simulink model "TST_EngBrk_ExhFlpCtl"  (R2016b)
settings: Solver=FixedStepDiscrete  StartTime=0.0  StopTime=simTime  FixedStep=sampleTime  RelTol=1e-3
values from neighbouring files (symbols this model uses):
  testCase = 1    [initTST_EngBrk_ExhFlpCtl_001.m]    (also in initTST_EngBrk_ExhFlpCtl_002.m = 2)
libraries: simulink x3
settings Model: Creator=WF305  LastModifiedBy=WF305
settings DebuggingCC: SignalRangeChecking=error

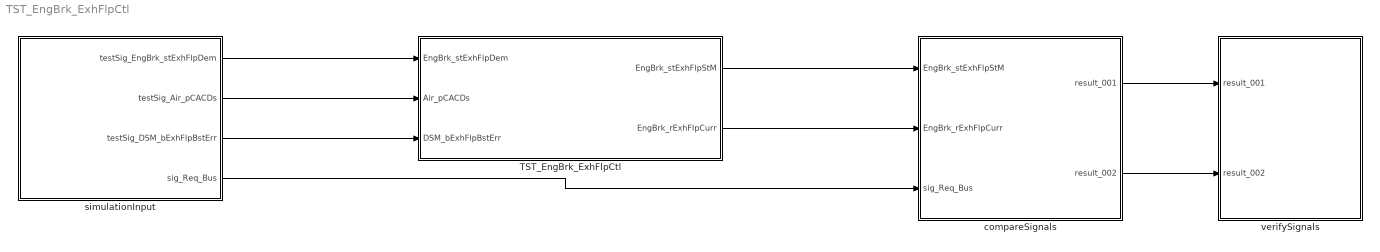
== system TST_EngBrk_ExhFlpCtl ==
  TST_EngBrk_ExhFlpCtl : Subsystem
  compareSignals : Subsystem
  simulationInput : Subsystem
  verifySignals : Subsystem
  wires:
  simulationInput/1(testSig_EngBrk_stExhFlpDem) -> TST_EngBrk_ExhFlpCtl/1(EngBrk_stExhFlpDem)
  simulationInput/2(testSig_Air_pCACDs) -> TST_EngBrk_ExhFlpCtl/2(Air_pCACDs)
  simulationInput/3(testSig_DSM_bExhFlpBstErr) -> TST_EngBrk_ExhFlpCtl/3(DSM_bExhFlpBstErr)
  TST_EngBrk_ExhFlpCtl/1(EngBrk_stExhFlpStM) -> compareSignals/1(EngBrk_stExhFlpStM)
  TST_EngBrk_ExhFlpCtl/2(EngBrk_rExhFlpCurr) -> compareSignals/2(EngBrk_rExhFlpCurr)
  simulationInput/4(sig_Req_Bus) -> compareSignals/3(sig_Req_Bus)
  compareSignals/1(result_001) -> verifySignals/1(result_001)
  compareSignals/2(result_002) -> verifySignals/2(result_002)

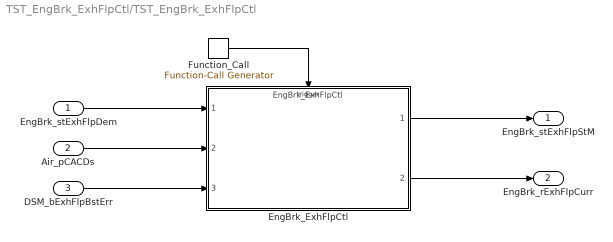
== system TST_EngBrk_ExhFlpCtl/TST_EngBrk_ExhFlpCtl ==
  EngBrk_stExhFlpDem : Inport
  Air_pCACDs : Inport  Port=2
  DSM_bExhFlpBstErr : Inport  Port=3
  EngBrk_ExhFlpCtl : ModelReference  ModelNameDialog=EngBrk_ExhFlpCtl  ModelReferenceVersion=1.4  TriggerPortName=function  TriggerPortTriggerType=function-call  TriggerPortStatesWhenEnabling=held
  Function_Call : simulink/Ports & Subsystems/Function-Call Generator  sample_time=sampleTime  numberOfIterations=1
  EngBrk_stExhFlpStM : Outport
  EngBrk_rExhFlpCurr : Outport  Port=2
  wires:
  Function_Call/1 -> EngBrk_ExhFlpCtl/Trigger
  EngBrk_stExhFlpDem/1 -> EngBrk_ExhFlpCtl/1
  Air_pCACDs/1 -> EngBrk_ExhFlpCtl/2
  DSM_bExhFlpBstErr/1 -> EngBrk_ExhFlpCtl/3
  EngBrk_ExhFlpCtl/1 -> EngBrk_stExhFlpStM/1
  EngBrk_ExhFlpCtl/2 -> EngBrk_rExhFlpCurr/1

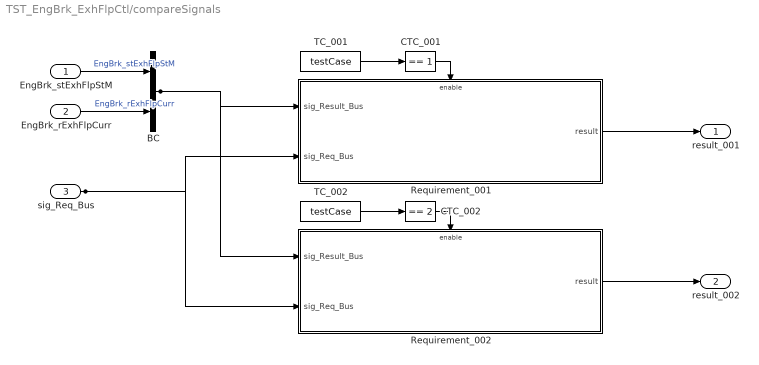
== system TST_EngBrk_ExhFlpCtl/compareSignals ==
  EngBrk_stExhFlpStM : Inport
  EngBrk_rExhFlpCurr : Inport  Port=2
  sig_Req_Bus : Inport  Port=3
  BC : BusCreator  Inputs=2
  CTC_001 : simulink/Logic and Bit Operations/Compare To Constant  relop===  const=1  OutDataTypeStr=boolean
  CTC_002 : simulink/Logic and Bit Operations/Compare To Constant  relop===  const=2  OutDataTypeStr=boolean
  Requirement_001 : Subsystem
  Requirement_002 : Subsystem
  TC_001 : Constant  Value=testCase
  TC_002 : Constant  Value=testCase
  result_001 : Outport
  result_002 : Outport  Port=2
  wires:
  EngBrk_stExhFlpStM/1 -> BC/1  "EngBrk_stExhFlpStM"
  EngBrk_rExhFlpCurr/1 -> BC/2  "EngBrk_rExhFlpCurr"
  TC_001/1 -> CTC_001/1
  CTC_001/1 -> Requirement_001/Enable
  sig_Req_Bus/1 -> Requirement_001/2(sig_Req_Bus), Requirement_002/2(sig_Req_Bus)
  BC/1 -> Requirement_001/1(sig_Result_Bus), Requirement_002/1(sig_Result_Bus)
  Requirement_001/1(result) -> result_001/1
  TC_002/1 -> CTC_002/1
  CTC_002/1 -> Requirement_002/Enable
  Requirement_002/1(result) -> result_002/1

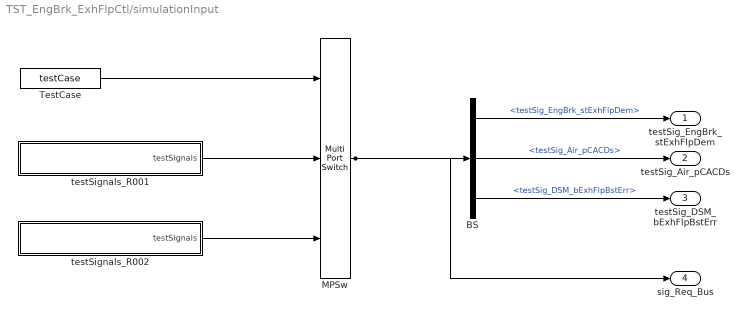
== system TST_EngBrk_ExhFlpCtl/simulationInput ==
  BS : BusSelector  OutputSignals=testSig_EngBrk_stExhFlpDem,testSig_Air_pCACDs,testSig_DSM_bExhFlpBstErr
  MPSw : MultiPortSwitch  Inputs=2  SaturateOnIntegerOverflow=on  InputSameDT=on
  TestCase : Constant  Value=testCase
  testSignals_R001 : Subsystem
  testSignals_R002 : Subsystem
  testSig_EngBrk_stExhFlpDem : Outport
  testSig_Air_pCACDs : Outport  Port=2
  testSig_DSM_bExhFlpBstErr : Outport  Port=3
  sig_Req_Bus : Outport  Port=4
  wires:
  BS/1 -> testSig_EngBrk_stExhFlpDem/1  "<testSig_EngBrk_stExhFlpDem>"
  BS/2 -> testSig_Air_pCACDs/1  "<testSig_Air_pCACDs>"
  BS/3 -> testSig_DSM_bExhFlpBstErr/1  "<testSig_DSM_bExhFlpBstErr>"
  MPSw/1 -> BS/1, sig_Req_Bus/1
  TestCase/1 -> MPSw/1
  testSignals_R001/1(testSignals) -> MPSw/2
  testSignals_R002/1(testSignals) -> MPSw/3

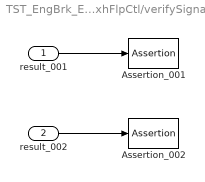
== system TST_EngBrk_ExhFlpCtl/verifySignals ==
  result_001 : Inport
  result_002 : Inport  Port=2
  Assertion_001 : Assertion  Enabled=off
  Assertion_002 : Assertion  Enabled=off
  wires:
  result_001/1 -> Assertion_001/1
  result_002/1 -> Assertion_002/1

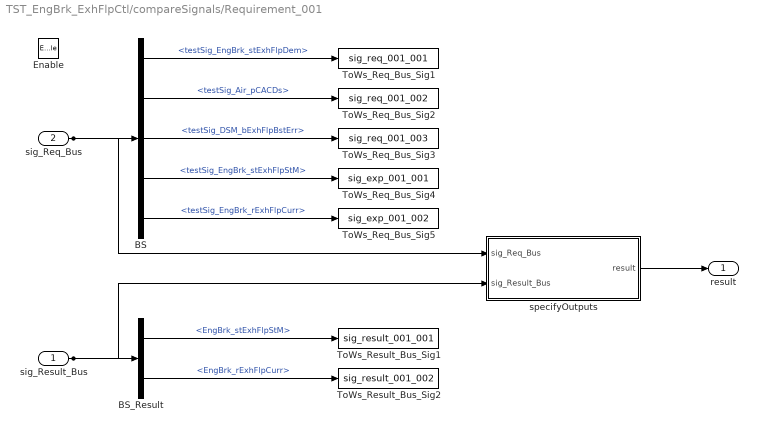
== system TST_EngBrk_ExhFlpCtl/compareSignals/Requirement_001 ==
  sig_Result_Bus : Inport
  sig_Req_Bus : Inport  Port=2
  Enable : EnablePort
  BS : BusSelector  OutputSignals=testSig_EngBrk_stExhFlpDem,testSig_Air_pCACDs,testSig_DSM_bExhFlpBstErr,testSig_EngBrk_stExhFlpStM,testSig_EngBrk_rExhFlpCurr
  BS_Result : BusSelector  OutputSignals=EngBrk_stExhFlpStM,EngBrk_rExhFlpCurr
  ToWs_Req_Bus_Sig1 : ToWorkspace  VariableName=sig_req_001_001  SaveFormat=Structure With Time
  ToWs_Req_Bus_Sig2 : ToWorkspace  VariableName=sig_req_001_002  SaveFormat=Structure With Time
  ToWs_Req_Bus_Sig3 : ToWorkspace  VariableName=sig_req_001_003  SaveFormat=Structure With Time
  ToWs_Req_Bus_Sig4 : ToWorkspace  VariableName=sig_exp_001_001  SaveFormat=Structure With Time
  ToWs_Req_Bus_Sig5 : ToWorkspace  VariableName=sig_exp_001_002  SaveFormat=Structure With Time
  ToWs_Result_Bus_Sig1 : ToWorkspace  VariableName=sig_result_001_001  SaveFormat=Structure With Time
  ToWs_Result_Bus_Sig2 : ToWorkspace  VariableName=sig_result_001_002  SaveFormat=Structure With Time
  specifyOutputs : Subsystem
  result : Outport
  wires:
  sig_Req_Bus/1 -> BS/1, specifyOutputs/1(sig_Req_Bus)
  BS/1 -> ToWs_Req_Bus_Sig1/1  "<testSig_EngBrk_stExhFlpDem>"
  BS/2 -> ToWs_Req_Bus_Sig2/1  "<testSig_Air_pCACDs>"
  BS/3 -> ToWs_Req_Bus_Sig3/1  "<testSig_DSM_bExhFlpBstErr>"
  BS/4 -> ToWs_Req_Bus_Sig4/1  "<testSig_EngBrk_stExhFlpStM>"
  BS/5 -> ToWs_Req_Bus_Sig5/1  "<testSig_EngBrk_rExhFlpCurr>"
  sig_Result_Bus/1 -> BS_Result/1, specifyOutputs/2(sig_Result_Bus)
  BS_Result/1 -> ToWs_Result_Bus_Sig1/1  "<EngBrk_stExhFlpStM>"
  BS_Result/2 -> ToWs_Result_Bus_Sig2/1  "<EngBrk_rExhFlpCurr>"
  specifyOutputs/1(result) -> result/1

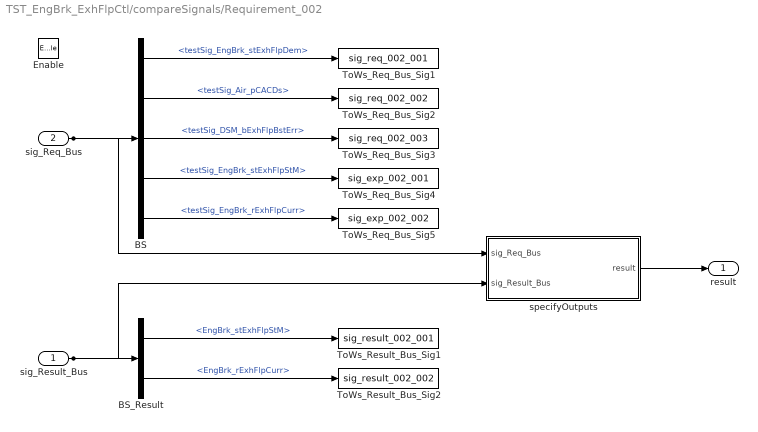
== system TST_EngBrk_ExhFlpCtl/compareSignals/Requirement_002 ==
  sig_Result_Bus : Inport
  sig_Req_Bus : Inport  Port=2
  Enable : EnablePort
  BS : BusSelector  OutputSignals=testSig_EngBrk_stExhFlpDem,testSig_Air_pCACDs,testSig_DSM_bExhFlpBstErr,testSig_EngBrk_stExhFlpStM,testSig_EngBrk_rExhFlpCurr
  BS_Result : BusSelector  OutputSignals=EngBrk_stExhFlpStM,EngBrk_rExhFlpCurr
  ToWs_Req_Bus_Sig1 : ToWorkspace  VariableName=sig_req_002_001  SaveFormat=Structure With Time
  ToWs_Req_Bus_Sig2 : ToWorkspace  VariableName=sig_req_002_002  SaveFormat=Structure With Time
  ToWs_Req_Bus_Sig3 : ToWorkspace  VariableName=sig_req_002_003  SaveFormat=Structure With Time
  ToWs_Req_Bus_Sig4 : ToWorkspace  VariableName=sig_exp_002_001  SaveFormat=Structure With Time
  ToWs_Req_Bus_Sig5 : ToWorkspace  VariableName=sig_exp_002_002  SaveFormat=Structure With Time
  ToWs_Result_Bus_Sig1 : ToWorkspace  VariableName=sig_result_002_001  SaveFormat=Structure With Time
  ToWs_Result_Bus_Sig2 : ToWorkspace  VariableName=sig_result_002_002  SaveFormat=Structure With Time
  specifyOutputs : Subsystem
  result : Outport
  wires:
  sig_Req_Bus/1 -> BS/1, specifyOutputs/1(sig_Req_Bus)
  BS/1 -> ToWs_Req_Bus_Sig1/1  "<testSig_EngBrk_stExhFlpDem>"
  BS/2 -> ToWs_Req_Bus_Sig2/1  "<testSig_Air_pCACDs>"
  BS/3 -> ToWs_Req_Bus_Sig3/1  "<testSig_DSM_bExhFlpBstErr>"
  BS/4 -> ToWs_Req_Bus_Sig4/1  "<testSig_EngBrk_stExhFlpStM>"
  BS/5 -> ToWs_Req_Bus_Sig5/1  "<testSig_EngBrk_rExhFlpCurr>"
  sig_Result_Bus/1 -> BS_Result/1, specifyOutputs/2(sig_Result_Bus)
  BS_Result/1 -> ToWs_Result_Bus_Sig1/1  "<EngBrk_stExhFlpStM>"
  BS_Result/2 -> ToWs_Result_Bus_Sig2/1  "<EngBrk_rExhFlpCurr>"
  specifyOutputs/1(result) -> result/1

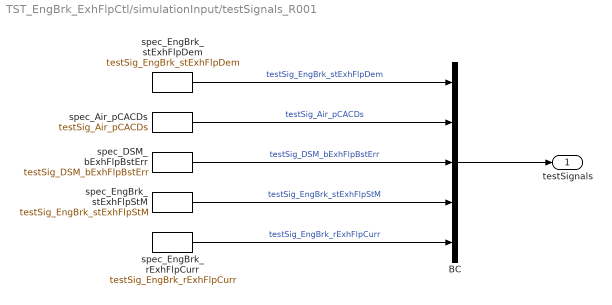
== system TST_EngBrk_ExhFlpCtl/simulationInput/testSignals_R001 ==
  BC : BusCreator  Inputs=5
  spec_Air_pCACDs : FromWorkspace  VariableName=testSig_Air_pCACDs  Interpolate=off  OutputAfterFinalValue=Holding final value
  spec_DSM_bExhFlpBstErr : FromWorkspace  VariableName=testSig_DSM_bExhFlpBstErr  Interpolate=off  OutputAfterFinalValue=Holding final value
  spec_EngBrk_rExhFlpCurr : FromWorkspace  VariableName=testSig_EngBrk_rExhFlpCurr  Interpolate=off  OutputAfterFinalValue=Holding final value
  spec_EngBrk_stExhFlpDem : FromWorkspace  VariableName=testSig_EngBrk_stExhFlpDem  Interpolate=off  OutputAfterFinalValue=Holding final value
  spec_EngBrk_stExhFlpStM : FromWorkspace  VariableName=testSig_EngBrk_stExhFlpStM  Interpolate=off  OutputAfterFinalValue=Holding final value
  testSignals : Outport
  wires:
  BC/1 -> testSignals/1
  spec_EngBrk_stExhFlpDem/1 -> BC/1  "testSig_EngBrk_stExhFlpDem"
  spec_Air_pCACDs/1 -> BC/2  "testSig_Air_pCACDs"
  spec_DSM_bExhFlpBstErr/1 -> BC/3  "testSig_DSM_bExhFlpBstErr"
  spec_EngBrk_stExhFlpStM/1 -> BC/4  "testSig_EngBrk_stExhFlpStM"
  spec_EngBrk_rExhFlpCurr/1 -> BC/5  "testSig_EngBrk_rExhFlpCurr"

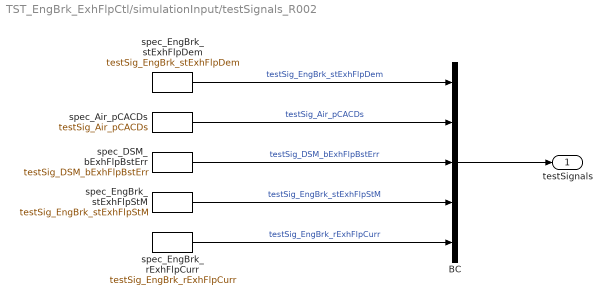
== system TST_EngBrk_ExhFlpCtl/simulationInput/testSignals_R002 ==
  BC : BusCreator  Inputs=5
  spec_Air_pCACDs : FromWorkspace  VariableName=testSig_Air_pCACDs  Interpolate=off  OutputAfterFinalValue=Holding final value
  spec_DSM_bExhFlpBstErr : FromWorkspace  VariableName=testSig_DSM_bExhFlpBstErr  Interpolate=off  OutputAfterFinalValue=Holding final value
  spec_EngBrk_rExhFlpCurr : FromWorkspace  VariableName=testSig_EngBrk_rExhFlpCurr  Interpolate=off  OutputAfterFinalValue=Holding final value
  spec_EngBrk_stExhFlpDem : FromWorkspace  VariableName=testSig_EngBrk_stExhFlpDem  Interpolate=off  OutputAfterFinalValue=Holding final value
  spec_EngBrk_stExhFlpStM : FromWorkspace  VariableName=testSig_EngBrk_stExhFlpStM  Interpolate=off  OutputAfterFinalValue=Holding final value
  testSignals : Outport
  wires:
  BC/1 -> testSignals/1
  spec_EngBrk_stExhFlpDem/1 -> BC/1  "testSig_EngBrk_stExhFlpDem"
  spec_Air_pCACDs/1 -> BC/2  "testSig_Air_pCACDs"
  spec_DSM_bExhFlpBstErr/1 -> BC/3  "testSig_DSM_bExhFlpBstErr"
  spec_EngBrk_stExhFlpStM/1 -> BC/4  "testSig_EngBrk_stExhFlpStM"
  spec_EngBrk_rExhFlpCurr/1 -> BC/5  "testSig_EngBrk_rExhFlpCurr"

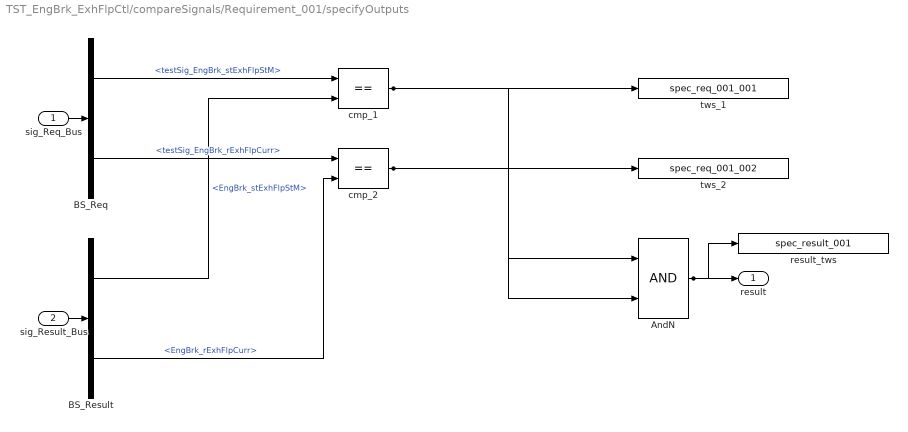
== system TST_EngBrk_ExhFlpCtl/compareSignals/Requirement_001/specifyOutputs ==
  sig_Req_Bus : Inport
  sig_Result_Bus : Inport  Port=2
  AndN : Logic
  BS_Req : BusSelector  OutputSignals=testSig_EngBrk_stExhFlpStM,testSig_EngBrk_rExhFlpCurr
  BS_Result : BusSelector  OutputSignals=EngBrk_stExhFlpStM,EngBrk_rExhFlpCurr
  cmp_1 : RelationalOperator  Operator===  RndMeth=Nearest  InputSameDT=on
  cmp_2 : RelationalOperator  Operator===  RndMeth=Nearest  InputSameDT=on
  result_tws : ToWorkspace  VariableName=spec_result_001
  tws_1 : ToWorkspace  VariableName=spec_req_001_001
  tws_2 : ToWorkspace  VariableName=spec_req_001_002
  result : Outport
  wires:
  sig_Req_Bus/1 -> BS_Req/1
  sig_Result_Bus/1 -> BS_Result/1
  AndN/1 -> result/1, result_tws/1
  BS_Req/1 -> cmp_1/1  "<testSig_EngBrk_stExhFlpStM>"
  BS_Result/1 -> cmp_1/2  "<EngBrk_stExhFlpStM>"
  cmp_1/1 -> tws_1/1, AndN/1
  BS_Req/2 -> cmp_2/1  "<testSig_EngBrk_rExhFlpCurr>"
  BS_Result/2 -> cmp_2/2  "<EngBrk_rExhFlpCurr>"
  cmp_2/1 -> tws_2/1, AndN/2

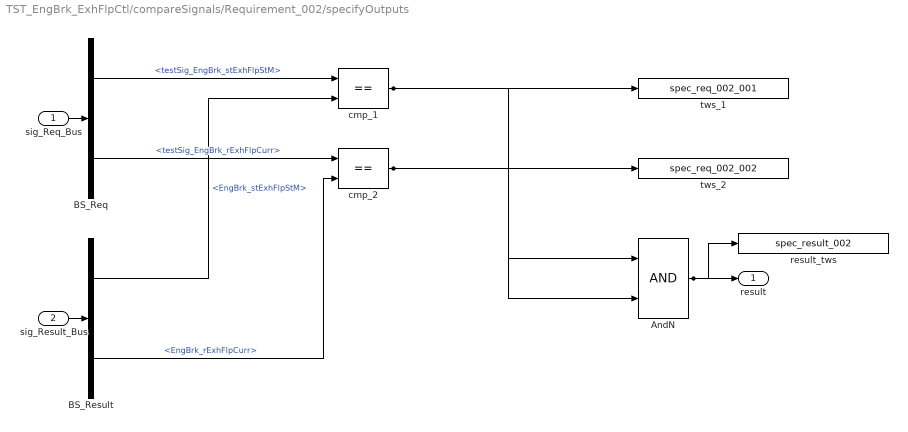
== system TST_EngBrk_ExhFlpCtl/compareSignals/Requirement_002/specifyOutputs ==
  sig_Req_Bus : Inport
  sig_Result_Bus : Inport  Port=2
  AndN : Logic
  BS_Req : BusSelector  OutputSignals=testSig_EngBrk_stExhFlpStM,testSig_EngBrk_rExhFlpCurr
  BS_Result : BusSelector  OutputSignals=EngBrk_stExhFlpStM,EngBrk_rExhFlpCurr
  cmp_1 : RelationalOperator  Operator===  RndMeth=Nearest  InputSameDT=on
  cmp_2 : RelationalOperator  Operator===  RndMeth=Nearest  InputSameDT=on
  result_tws : ToWorkspace  VariableName=spec_result_002
  tws_1 : ToWorkspace  VariableName=spec_req_002_001
  tws_2 : ToWorkspace  VariableName=spec_req_002_002
  result : Outport
  wires:
  sig_Req_Bus/1 -> BS_Req/1
  sig_Result_Bus/1 -> BS_Result/1
  AndN/1 -> result/1, result_tws/1
  BS_Req/1 -> cmp_1/1  "<testSig_EngBrk_stExhFlpStM>"
  BS_Result/1 -> cmp_1/2  "<EngBrk_stExhFlpStM>"
  cmp_1/1 -> tws_1/1, AndN/1
  BS_Req/2 -> cmp_2/1  "<testSig_EngBrk_rExhFlpCurr>"
  BS_Result/2 -> cmp_2/2  "<EngBrk_rExhFlpCurr>"
  cmp_2/1 -> tws_2/1, AndN/2
